simulink model "simex2"  (R2023b)
settings: Solver=VariableStepAuto  StartTime=0.0  StopTime=10  RelTol=1e-3
undefined symbols (not defined in the file or in its folder): DiscIntNeverNeededParam
libraries: simulink x6
settings Model: PacingRate=0.220000  Creator=Vinar  LastModifiedBy=majko
settings OptimizationCC: ReuseModelBlockBuffer=off

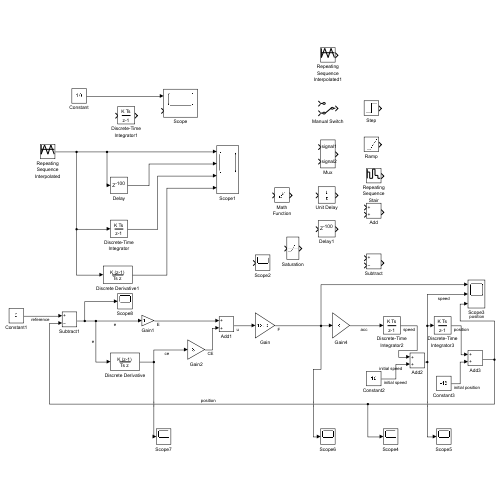
[thumbnail: Simulink's stored preview of the top-level diagram]
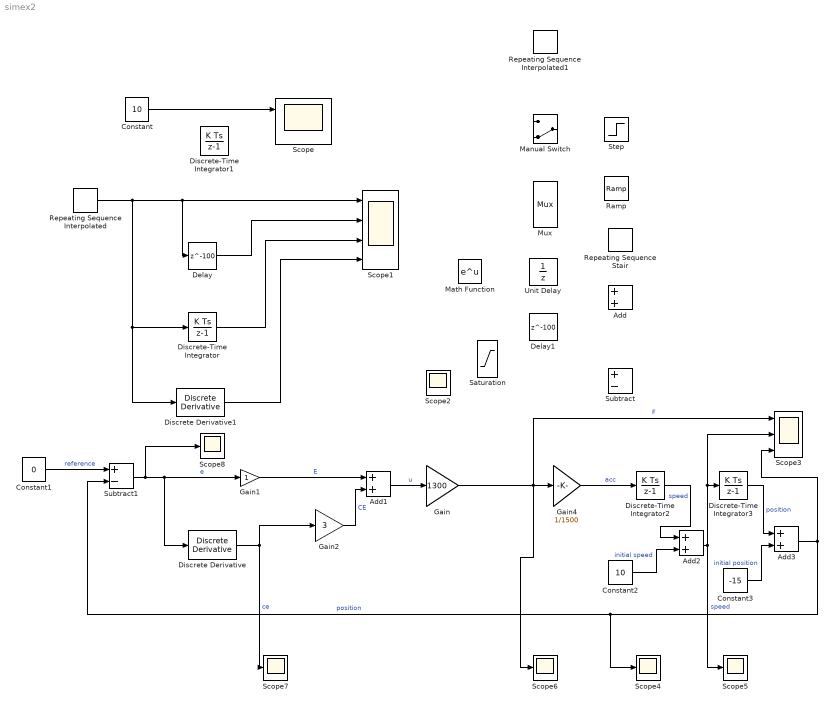
== system simex2 ==
  Add{,1..3} (4 alike) : Sum
  Constant : Constant  Value=10  SampleTime=0
  Constant1 : Constant  Value=0
  Constant2 : Constant  Value=10
  Constant3 : Constant  Value=-15
  Delay : Delay  DelayLength=100  InitialCondition=-100  SampleTime=0.1
  Delay1 : Delay  DelayLength=100  InitialCondition=-100  SampleTime=0.1
  Discrete Derivative : simulink/Discrete/Discrete Derivative  gainval=1.0  ICPrevScaledInput=150  InputProcessing=Columns as channels (frame based)  OutMin=[]  OutMax=[]  OutDataType=fixdt(1, 16)  OutScaling=2^-10  DoSatur=off
  Discrete Derivative1 : simulink/Discrete/Discrete Derivative  gainval=1.0  ICPrevScaledInput=-1000  OutMin=[]  OutMax=[]  OutDataType=fixdt(1, 16)  OutScaling=2^-10  DoSatur=off
  Discrete-Time Integrator : DiscreteIntegrator  SampleTime=0.1  ICPrevOutput=DiscIntNeverNeededParam  ICPrevScaledInput=DiscIntNeverNeededParam
  Discrete-Time Integrator1 : DiscreteIntegrator  ICPrevOutput=DiscIntNeverNeededParam  ICPrevScaledInput=DiscIntNeverNeededParam
  Discrete-Time Integrator2 : DiscreteIntegrator  SampleTime=0.1  ICPrevOutput=DiscIntNeverNeededParam  ICPrevScaledInput=DiscIntNeverNeededParam
  Discrete-Time Integrator3 : DiscreteIntegrator  SampleTime=0.1  ICPrevOutput=DiscIntNeverNeededParam  ICPrevScaledInput=DiscIntNeverNeededParam
  Gain : Gain  Gain=1300
  Gain1 : Gain
  Gain2 : Gain  Gain=3
  Gain4 : Gain  Gain=1/1500
  Manual Switch : ManualSwitch  CurrentSetting=0
  Math Function : Math
  Mux : Mux  Inputs=2
      settings: DisplayOption=signals
  Ramp : simulink/Sources/Ramp  slope=1  start=0  InitialOutput=0
  Repeating Sequence Interpolated : simulink/Sources/Repeating Sequence Interpolated  OutValues=[-100 100 -100 100 -100].'  TimeValues=[0 50 100 150 200].'  LookUpMeth=Interpolation-Use End Values  tsamp=0.1  OutMin=[]  OutMax=[]  OutDataTypeStr=double  OutputDataTypeScalingMode=double  OutDataType=fixdt(0,8)  OutScaling=2^-10
  Repeating Sequence Interpolated1 : simulink/Sources/Repeating Sequence Interpolated  OutValues=[-100 100 -100 100 -100].'  TimeValues=[0 50 100 150 200].'  LookUpMeth=Interpolation-Use End Values  tsamp=0.1  OutMin=[]  OutMax=[]  OutDataTypeStr=double  OutputDataTypeScalingMode=double  OutDataType=fixdt(0,8)  OutScaling=2^-10
  Repeating Sequence Stair : simulink/Sources/Repeating Sequence Stair  OutValues=[3 1 4 2 1].'  tsamp=-1  OutMin=[]  OutMax=[]  OutDataTypeStr=double  OutputDataTypeScalingMode=double  OutDataType=fixdt(0,8)  ConRadixGroup=Best Precision: Vector-wise  OutScaling=2^-12
  Saturation : Saturate  UpperLimit=0  LowerLimit=-14000
  Scope : Scope  NumInputPorts=2
  Scope1 : Scope  NumInputPorts=4
  Scope{2,4..8} (6 alike) : Scope
  Scope3 : Scope  NumInputPorts=3
  Step : Step  SampleTime=0
  Subtract : Sum  Inputs=+-
  Subtract1 : Sum  Inputs=+-
  Unit Delay : UnitDelay  SampleTime=-1  HasFrameUpgradeWarning=on
  wires:
  Delay/1 -> Scope1/2
  Repeating Sequence Interpolated/1 -> Discrete Derivative1/1, Discrete-Time Integrator/1, Delay/1, Scope1/1
  Discrete-Time Integrator/1 -> Scope1/3
  Constant/1 -> Scope/1
  Discrete Derivative1/1 -> Scope1/4
  Constant1/1 -> Subtract1/1  "reference"
  Subtract1/1 -> Scope8/1, Discrete Derivative/1, Gain1/1  "e"
  Gain1/1 -> Add1/1  "E"
  Discrete Derivative/1 -> Scope7/1, Gain2/1  "ce"
  Add1/1 -> Gain/1  "u"
  Gain4/1 -> Discrete-Time Integrator2/1  "acc"
  Gain/1 -> Scope6/1, Scope3/1, Gain4/1  "F"
  Discrete-Time Integrator2/1 -> Add2/1  "speed"
  Add2/1 -> Scope3/2, Discrete-Time Integrator3/1, Scope5/1  "speed"
  Discrete-Time Integrator3/1 -> Add3/1  "position"
  Add3/1 -> Scope4/1, Subtract1/2, Scope3/3  "position"
  Constant2/1 -> Add2/2  "initial speed"
  Constant3/1 -> Add3/2  "initial position"
  Gain2/1 -> Add1/2  "CE"
